simulink model "refSuntest"  (R2018a)
settings: Solver=FixedStepDiscrete  StartTime=0  StopTime=init.S_T*20  FixedStep=1000  RelTol=1e-3
undefined symbols (not defined in the file or in its folder): init, km, s
libraries: dspstat3 x1, vrlib x1, aerolibcelestial x1
settings Model: Creator=nathan  LastModifiedBy=nathan

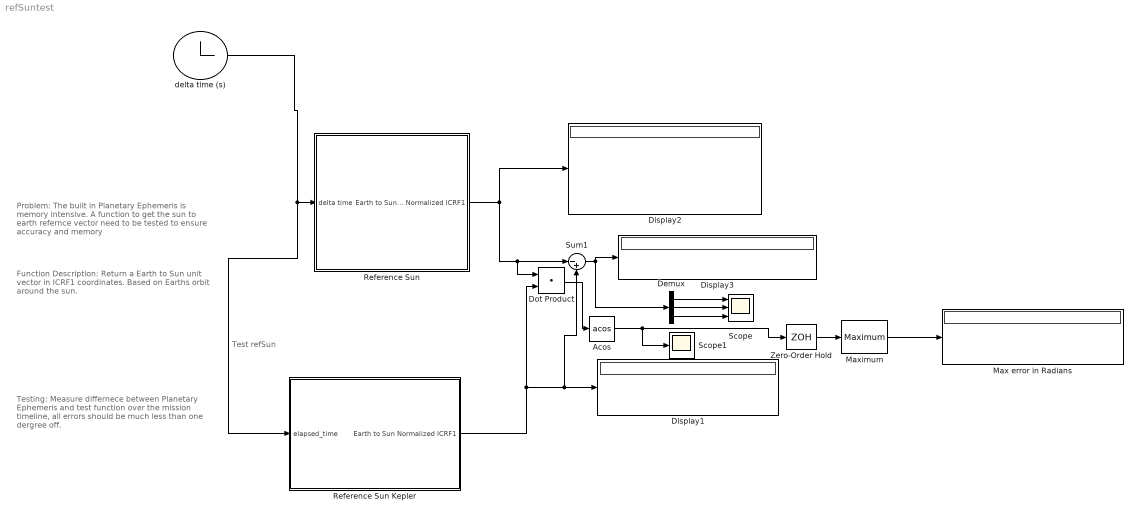
== system refSuntest ==
  note: Function Description:
      | Return a Earth to Sun unit vector in ICRF1 coordinates.
      | Based on Earths orbit around the sun.
  note: Problem:
      | The built in Planetary Ephemeris is memory intensive. A function to get the sun to earth refernce vector need to be tested to ensure accuracy and memory
  note: Testing:
      | Measure differnece between Planetary Ephemeris and test function over the mission timeline, all errors should be much less than one dergree off.
  note: Test refSun
  Acos : Trigonometry  Operator=acos
  Demux : Demux  Outputs=3
  Display1 : Display
  Display2 : Display
  Display3 : Display
  Dot Product : DotProduct  InputSameDT=on  OutDataTypeStr=Inherit: Inherit via internal rule
  Max error in Radians : Display
  Maximum : dspstat3/Maximum  operation=maximum  fcn=Running  indexBase=One  operateOver=Entire input  Dimension=1  reset=None  roiEnable=off  roiType=Rectangles  roiPortion=Entire ROI  roiOutput=Individual statistics for each ROI  roiFlag=off  roundingMode=Floor  overflowMode=off  accumDataTypeStr=Inherit: Same as product output  accumLastDataTypeStr=Inherit: Same as product output
  "Reference Sun " : Subsystem
  Reference Sun Kepler : Subsystem  mask{tp=init.S_tp, yearT=init.S_T, e=init.S_e, q=init.S_q}
      mask prompts: tp "tp(double): delta time when the earth is at perihelion in seconds"; yearT "yearT(positive double): earths orbital period in seconds"; e "e(positive double): eccentricity of earths orbit"; q "q(quaterinion): quaternion to rotate from SUN to ICRF. SUN is a frame with z axis normal to earths orbital plane and x axis vector from sun to perihelion"
      mask DialogControl DescTextVar Prompt: Return the normalized vector from earth to sun in ECI. A very simple model of the earth orbiting around the sun in a keplerian orbit.
  Scope : Scope  NumInputPorts=3
  Scope1 : Scope
  Sum1 : Sum  Inputs=|-+
  Zero-Order Hold : ZeroOrderHold  SampleTime=-1
  delta time (s) : Clock
  wires:
  delta time (s)/1 -> Reference Sun Kepler/1(elapsed_time), "Reference Sun "/1(delta time)
  "Reference Sun "/1(Earth to Sun Normalized ICRF1) -> Display2/1, Dot Product/1, Sum1/1
  Sum1/1 -> Demux/1, Display3/1
  Demux/1 -> Scope/1
  Demux/2 -> Scope/2
  Demux/3 -> Scope/3
  Dot Product/1 -> Acos/1
  Acos/1 -> Scope1/1, Zero-Order Hold/1
  Maximum/1 -> Max error in Radians/1
  Zero-Order Hold/1 -> Maximum/1
  Reference Sun Kepler/1(Earth to Sun Normalized ICRF1) -> Dot Product/2, Sum1/2, Display1/1

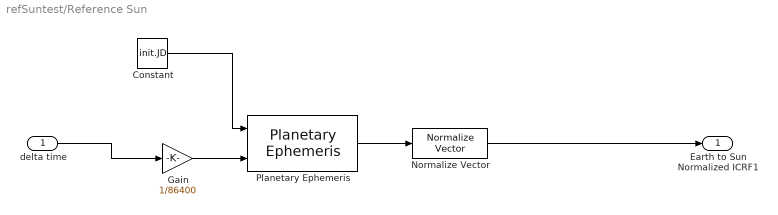
== system refSuntest/Reference Sun  ==
  delta time : Inport
  Constant : Constant  Value=init.JD
  Gain : Gain  Gain=1/86400
  Normalize Vector : vrlib/Utilities/Normalize Vector  maxzero=0
      settings: SourceProductName=Simulink 3D Animation  SourceProductBaseCode=VR
  Planetary Ephemeris : aerolibcelestial/Planetary Ephemeris  kmflag=km,km/s  epochflag=T0 and elapsed Julian time  de=DE405  nCenter=Earth  nTarget=Sun  errorflag=Error  velflag=off
      settings: SourceProductName=Aerospace Blockset  SourceProductBaseCode=AE
  Earth to Sun Normalized ICRF1 : Outport
  wires:
  Normalize Vector/1 -> Earth to Sun Normalized ICRF1/1
  Planetary Ephemeris/1 -> Normalize Vector/1
  delta time/1 -> Gain/1
  Constant/1 -> Planetary Ephemeris/1
  Gain/1 -> Planetary Ephemeris/2

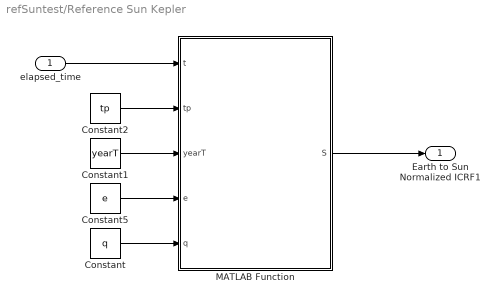
== system refSuntest/Reference Sun Kepler ==
  elapsed_time : Inport
  Constant : Constant  Value=q
  Constant1 : Constant  Value=yearT
  Constant2 : Constant  Value=tp
  Constant5 : Constant  Value=e
  MATLAB Function : MATLAB Function  TreatAsAtomicUnit=on
  Earth to Sun Normalized ICRF1 : Outport
  wires:
  MATLAB Function/1(S) -> Earth to Sun Normalized ICRF1/1
  Constant1/1 -> MATLAB Function/3(yearT)
  elapsed_time/1 -> MATLAB Function/1(t)
  Constant5/1 -> MATLAB Function/4(e)
  Constant2/1 -> MATLAB Function/2(tp)
  Constant/1 -> MATLAB Function/5(q)

== matlab function refSuntest/Reference Sun Kepler/MATLAB Function ==
  data: t input; S output; tp input; yearT input; e input; q input
function S = fcn(t,tp,yearT,e,q)
%sds
S= refSunK(t,tp,yearT,e,q);
